simulink model "Simulink_multiterminal_HVDC_grid"  (R2016a)
settings: Solver=ode4  StartTime=0.0  StopTime=tsimul  FixedStep=1e-5  MaxStep=1e-4  RelTol=1e-5
values from neighbouring files (symbols this model uses):
  c = 0.1616*(10^-6)    (= 1.616e-07)    [Parameters_multiterminal_HVDC_grid.m]
  Cconv = 1.5*(10^-4)    (= 0.00015)    [Parameters_multiterminal_HVDC_grid.m]
  d1 = 230    [Parameters_multiterminal_HVDC_grid.m]
  d2 = 75    [Parameters_multiterminal_HVDC_grid.m]
  d3 = 217    [Parameters_multiterminal_HVDC_grid.m]
  E2ref = 640000    [Parameters_multiterminal_HVDC_grid.m]
  Kp = 0.0017    [Parameters_multiterminal_HVDC_grid.m]
  l1 = 0.2644*(10^-3)    (= 0.0002644)    [Parameters_multiterminal_HVDC_grid.m]
  l2 = 7.2865*(10^-3)    (= 0.0072865)    [Parameters_multiterminal_HVDC_grid.m]
  l3 = 3.6198*(10^-3)    (= 0.0036198)    [Parameters_multiterminal_HVDC_grid.m]
  Ll = 0.1956    [Parameters_multiterminal_HVDC_grid.m]
  Qref = 0    [Parameters_multiterminal_HVDC_grid.m]
  r1 = 0.1265    [Parameters_multiterminal_HVDC_grid.m]
  r2 = 0.1504    [Parameters_multiterminal_HVDC_grid.m]
  r3 = 0.0178    [Parameters_multiterminal_HVDC_grid.m]
  Rg = (1/g)    (= 9852216.74877)    [Parameters_multiterminal_HVDC_grid.m]
  rl = 3.072    [Parameters_multiterminal_HVDC_grid.m]
  tau = 0.001    [Parameters_multiterminal_HVDC_grid.m]
  taupll = 0.0045    [Parameters_multiterminal_HVDC_grid.m]
  Uab = 320000    [Parameters_multiterminal_HVDC_grid.m]
  Vdc = 640000    [Parameters_multiterminal_HVDC_grid.m]
undefined symbols (not defined in the file or in its folder): Kpdc
libraries: powerlib x115, simulink x4
(part 1 of 2)
settings Model: Creator=usuario  LastModifiedBy=usuario
settings DataIOCC: SaveFormat=StructureWithTime
settings DebuggingCC: AllowSymbolicDim=off
settings HardwareCC: ProdWordSize=32  ProdHWDeviceType=Specified

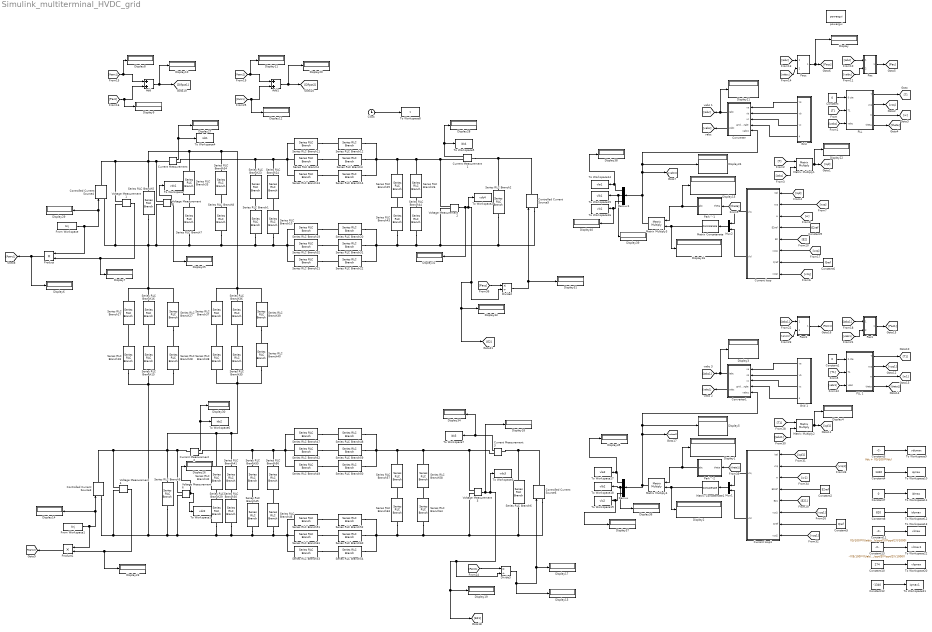
== system Simulink_multiterminal_HVDC_grid ==
  Add : Sum
  Add1 : Sum
  Clock : Clock
  Constant : Constant  Value=0
  Constant1 : Constant  Value=0
  Constant10 : Constant  Value=274
  Constant11 : Constant  Value=((5/100)*((Uab/sqrt(3))*sqrt(2))/1000)+(((Uab/sqrt(3))*sqrt(2))/1000)
  Constant12 : Constant  Value=-1340
  Constant13 : Constant  Value=-(((5/100)*((Uab/sqrt(3))*sqrt(2))/1000)+(((Uab/sqrt(3))*sqrt(2))/1000))
  Constant2 : Constant  Value=E2ref
  Constant3 : Constant  Value=Vdc + ((5/100)*Vdc)
  Constant4 : Constant  Value=1340
  Constant5 : Constant  Value=Qref
  Constant6 : Constant  Value=Qref
  Constant7 : Constant  Value=0
  Constant8 : Constant  Value=820
  Constant9 : Constant  Value=E2ref
  Controlled Current Source{3..6} (4 alike) : powerlib/Electrical Sources/Controlled Current Source  Initialize=on  Source_Type=AC  Amplitude=0  Phase=0  Frequency=0  Measurements=None
  Converter : Subsystem
  Converter1 : Subsystem
  Current Measurement{,1..3} (4 alike) : powerlib/Measurements/Current Measurement  PhasorSimulation=off  OutputType=Complex  PSBequivalent=0
  Current loop : Subsystem
  Current loop1 : Subsystem
  Demux : Demux  Outputs=3
  Demux1 : Demux  Outputs=3
  Display{,1..40} (41 alike) : Display
  Divide2 : Product  Inputs=*/
  Divide3 : Product  Inputs=*/
  From Workspace : FromWorkspace  VariableName=Iinj  SampleTime=0
  From Workspace1 : FromWorkspace  VariableName=Iinj  SampleTime=0
  "Grid " : Subsystem
  Grid 1 : Subsystem
  Matrix Concatenate : Concatenate  NumInputs=1  Mode=Multidimensional array  ConcatenateDimension=2
  Matrix Concatenate1 : Concatenate  NumInputs=1  Mode=Multidimensional array  ConcatenateDimension=2
  Matrix Multiply{1..4} (4 alike) : Product  Multiplication=Matrix(*)
  Mux1 : Mux  Inputs=2
  Mux2 : Mux  Inputs=2
  "PLL " : Subsystem
  PLL 1 : Subsystem
  Pac : Subsystem
  Pac1 : Subsystem
  Pacc : Subsystem
  Pacc1 : Subsystem
  Park^-1 : Subsystem
  Park^-2 : Subsystem
  Product : Product
  Product1 : Product
  Series RLC Branch{1,23,25,43} (4 alike) : powerlib/Elements/Series RLC Branch  LConnTagsString=__new0  RConnTagsString=__new0  BranchType=R  Resistance=(Rg/d1)*(1/2)  Inductance=1e-3  SetiL0=off  InitialCurrent=0  Capacitance=1e-6  Setx0=off  InitialVoltage=0  Measurements=None
  Series RLC Branch10 : powerlib/Elements/Series RLC Branch  LConnTagsString=__new0  RConnTagsString=__new0  BranchType=C  Resistance=0  Inductance=0  SetiL0=off  InitialCurrent=0  Capacitance=(c/2)*d1  Setx0=on  InitialVoltage=Vdc  Measurements=None
  Series RLC Branch11 : powerlib/Elements/Series RLC Branch  LConnTagsString=__new0  RConnTagsString=__new0  BranchType=R  Resistance=r1*d1  Inductance=1e-3  SetiL0=off  InitialCurrent=0  Capacitance=1e-6  Setx0=off  InitialVoltage=0  Measurements=None
  Series RLC Branch12 : powerlib/Elements/Series RLC Branch  LConnTagsString=__new0  RConnTagsString=__new0  BranchType=L  Resistance=1  Inductance=l1*d1  SetiL0=off  InitialCurrent=0  Capacitance=1e-6  Setx0=off  InitialVoltage=0  Measurements=None
  Series RLC Branch13 : powerlib/Elements/Series RLC Branch  LConnTagsString=__new0  RConnTagsString=__new0  BranchType=R  Resistance=r3*d1  Inductance=1e-3  SetiL0=off  InitialCurrent=0  Capacitance=1e-6  Setx0=off  InitialVoltage=0  Measurements=None
  Series RLC Branch14 : powerlib/Elements/Series RLC Branch  LConnTagsString=__new0  RConnTagsString=__new0  BranchType=L  Resistance=1  Inductance=l3*d1  SetiL0=off  InitialCurrent=0  Capacitance=1e-6  Setx0=off  InitialVoltage=0  Measurements=None
  Series RLC Branch15 : powerlib/Elements/Series RLC Branch  LConnTagsString=__new0  RConnTagsString=__new0  BranchType=L  Resistance=1  Inductance=l2*d2  SetiL0=off  InitialCurrent=0  Capacitance=1e-6  Setx0=off  InitialVoltage=0  Measurements=None
  Series RLC Branch16 : powerlib/Elements/Series RLC Branch  LConnTagsString=__new0  RConnTagsString=__new0  BranchType=R  Resistance=r2*d2  Inductance=1e-3  SetiL0=off  InitialCurrent=0  Capacitance=1e-6  Setx0=off  InitialVoltage=0  Measurements=None
  Series RLC Branch17 : powerlib/Elements/Series RLC Branch  LConnTagsString=__new0  RConnTagsString=__new0  BranchType=R  Resistance=r1*d2  Inductance=1e-3  SetiL0=off  InitialCurrent=0  Capacitance=1e-6  Setx0=off  InitialVoltage=0  Measurements=None
  Series RLC Branch18 : powerlib/Elements/Series RLC Branch  LConnTagsString=__new0  RConnTagsString=__new0  BranchType=L  Resistance=1  Inductance=l1*d2  SetiL0=off  InitialCurrent=0  Capacitance=1e-6  Setx0=off  InitialVoltage=0  Measurements=None
  Series RLC Branch19 : powerlib/Elements/Series RLC Branch  LConnTagsString=__new0  RConnTagsString=__new0  BranchType=R  Resistance=r1*d1  Inductance=1e-3  SetiL0=off  InitialCurrent=0  Capacitance=1e-6  Setx0=off  InitialVoltage=0  Measurements=None
  Series RLC Branch2 : powerlib/Elements/Series RLC Branch  LConnTagsString=__new0  RConnTagsString=__new0  BranchType=C  Resistance=0  Inductance=0  SetiL0=off  InitialCurrent=0  Capacitance=Cconv  Setx0=on  InitialVoltage=Vdc  Measurements=None
  Series RLC Branch20 : powerlib/Elements/Series RLC Branch  LConnTagsString=__new0  RConnTagsString=__new0  BranchType=L  Resistance=1  Inductance=l1*d1  SetiL0=off  InitialCurrent=0  Capacitance=1e-6  Setx0=off  InitialVoltage=0  Measurements=None
  Series RLC Branch21 : powerlib/Elements/Series RLC Branch  LConnTagsString=__new0  RConnTagsString=__new0  BranchType=R  Resistance=r3*d1  Inductance=1e-3  SetiL0=off  InitialCurrent=0  Capacitance=1e-6  Setx0=off  InitialVoltage=0  Measurements=None
  Series RLC Branch22 : powerlib/Elements/Series RLC Branch  LConnTagsString=__new0  RConnTagsString=__new0  BranchType=L  Resistance=1  Inductance=l3*d1  SetiL0=off  InitialCurrent=0  Capacitance=1e-6  Setx0=off  InitialVoltage=0  Measurements=None
  Series RLC Branch24 : powerlib/Elements/Series RLC Branch  LConnTagsString=__new0  RConnTagsString=__new0  BranchType=C  Resistance=0  Inductance=0  SetiL0=off  InitialCurrent=0  Capacitance=(c/2)*d1  Setx0=on  InitialVoltage=Vdc  Measurements=None
  Series RLC Branch26 : powerlib/Elements/Series RLC Branch  LConnTagsString=__new0  RConnTagsString=__new0  BranchType=C  Resistance=0  Inductance=0  SetiL0=off  InitialCurrent=0  Capacitance=(c/2)*d1  Setx0=on  InitialVoltage=Vdc  Measurements=None
  Series RLC Branch27 : powerlib/Elements/Series RLC Branch  LConnTagsString=__new0  RConnTagsString=__new0  BranchType=R  Resistance=r3*d2  Inductance=1e-3  SetiL0=off  InitialCurrent=0  Capacitance=1e-6  Setx0=off  InitialVoltage=0  Measurements=None
  Series RLC Branch28 : powerlib/Elements/Series RLC Branch  LConnTagsString=__new0  RConnTagsString=__new0  BranchType=L  Resistance=1  Inductance=l3*d2  SetiL0=off  InitialCurrent=0  Capacitance=1e-6  Setx0=off  InitialVoltage=0  Measurements=None
  Series RLC Branch29 : powerlib/Elements/Series RLC Branch  LConnTagsString=__new0  RConnTagsString=__new0  BranchType=C  Resistance=0  Inductance=0  SetiL0=off  InitialCurrent=0  Capacitance=(c/2)*d2  Setx0=on  InitialVoltage=Vdc  Measurements=None
  Series RLC Branch3 : powerlib/Elements/Series RLC Branch  LConnTagsString=__new0  RConnTagsString=__new0  BranchType=L  Resistance=1  Inductance=l2*d1  SetiL0=off  InitialCurrent=0  Capacitance=1e-6  Setx0=off  InitialVoltage=0  Measurements=None
  Series RLC Branch{7,30,33,41} (4 alike) : powerlib/Elements/Series RLC Branch  LConnTagsString=__new0  RConnTagsString=__new0  BranchType=R  Resistance=(Rg/d2)*(1/2)  Inductance=1e-3  SetiL0=off  InitialCurrent=0  Capacitance=1e-6  Setx0=off  InitialVoltage=0  Measurements=None
  Series RLC Branch31 : powerlib/Elements/Series RLC Branch  LConnTagsString=__new0  RConnTagsString=__new0  BranchType=L  Resistance=1  Inductance=l2*d1  SetiL0=off  InitialCurrent=0  Capacitance=1e-6  Setx0=off  InitialVoltage=0  Measurements=None
  Series RLC Branch32 : powerlib/Elements/Series RLC Branch  LConnTagsString=__new0  RConnTagsString=__new0  BranchType=R  Resistance=r2*d1  Inductance=1e-3  SetiL0=off  InitialCurrent=0  Capacitance=1e-6  Setx0=off  InitialVoltage=0  Measurements=None
  Series RLC Branch34 : powerlib/Elements/Series RLC Branch  LConnTagsString=__new0  RConnTagsString=__new0  BranchType=C  Resistance=0  Inductance=0  SetiL0=off  InitialCurrent=0  Capacitance=(c/2)*d2  Setx0=on  InitialVoltage=Vdc  Measurements=None
  Series RLC Branch35 : powerlib/Elements/Series RLC Branch  LConnTagsString=__new0  RConnTagsString=__new0  BranchType=L  Resistance=1  Inductance=l2*d2  SetiL0=off  InitialCurrent=0  Capacitance=1e-6  Setx0=off  InitialVoltage=0  Measurements=None
  Series RLC Branch36 : powerlib/Elements/Series RLC Branch  LConnTagsString=__new0  RConnTagsString=__new0  BranchType=R  Resistance=r2*d2  Inductance=1e-3  SetiL0=off  InitialCurrent=0  Capacitance=1e-6  Setx0=off  InitialVoltage=0  Measurements=None
  Series RLC Branch37 : powerlib/Elements/Series RLC Branch  LConnTagsString=__new0  RConnTagsString=__new0  BranchType=R  Resistance=r1*d2  Inductance=1e-3  SetiL0=off  InitialCurrent=0  Capacitance=1e-6  Setx0=off  InitialVoltage=0  Measurements=None
  Series RLC Branch38 : powerlib/Elements/Series RLC Branch  LConnTagsString=__new0  RConnTagsString=__new0  BranchType=L  Resistance=1  Inductance=l1*d2  SetiL0=off  InitialCurrent=0  Capacitance=1e-6  Setx0=off  InitialVoltage=0  Measurements=None
  Series RLC Branch39 : powerlib/Elements/Series RLC Branch  LConnTagsString=__new0  RConnTagsString=__new0  BranchType=R  Resistance=r3*d2  Inductance=1e-3  SetiL0=off  InitialCurrent=0  Capacitance=1e-6  Setx0=off  InitialVoltage=0  Measurements=None
  Series RLC Branch4 : powerlib/Elements/Series RLC Branch  LConnTagsString=__new0  RConnTagsString=__new0  BranchType=R  Resistance=r2*d1  Inductance=1e-3  SetiL0=off  InitialCurrent=0  Capacitance=1e-6  Setx0=off  InitialVoltage=0  Measurements=None
  Series RLC Branch40 : powerlib/Elements/Series RLC Branch  LConnTagsString=__new0  RConnTagsString=__new0  BranchType=L  Resistance=1  Inductance=l3*d2  SetiL0=off  InitialCurrent=0  Capacitance=1e-6  Setx0=off  InitialVoltage=0  Measurements=None
  Series RLC Branch42 : powerlib/Elements/Series RLC Branch  LConnTagsString=__new0  RConnTagsString=__new0  BranchType=C  Resistance=0  Inductance=0  SetiL0=off  InitialCurrent=0  Capacitance=(c/2)*d2  Setx0=on  InitialVoltage=Vdc  Measurements=None
  Series RLC Branch44 : powerlib/Elements/Series RLC Branch  LConnTagsString=__new0  RConnTagsString=__new0  BranchType=C  Resistance=0  Inductance=0  SetiL0=off  InitialCurrent=0  Capacitance=(c/2)*d1  Setx0=off  InitialVoltage=Vdc  Measurements=None
  Series RLC Branch{45,55,57,63} (4 alike) : powerlib/Elements/Series RLC Branch  LConnTagsString=__new0  RConnTagsString=__new0  BranchType=R  Resistance=(Rg/d3)*(1/2)  Inductance=1e-3  SetiL0=off  InitialCurrent=0  Capacitance=1e-6  Setx0=off  InitialVoltage=0  Measurements=None
  Series RLC Branch46 : powerlib/Elements/Series RLC Branch  LConnTagsString=__new0  RConnTagsString=__new0  BranchType=C  Resistance=0  Inductance=0  SetiL0=off  InitialCurrent=0  Capacitance=(c/2)*d3  Setx0=on  InitialVoltage=Vdc  Measurements=None
  Series RLC Branch47 : powerlib/Elements/Series RLC Branch  LConnTagsString=__new0  RConnTagsString=__new0  BranchType=R  Resistance=r1*d3  Inductance=1e-3  SetiL0=off  InitialCurrent=0  Capacitance=1e-6  Setx0=off  InitialVoltage=0  Measurements=None
  Series RLC Branch48 : powerlib/Elements/Series RLC Branch  LConnTagsString=__new0  RConnTagsString=__new0  BranchType=L  Resistance=1  Inductance=l1*d3  SetiL0=off  InitialCurrent=0  Capacitance=1e-6  Setx0=off  InitialVoltage=0  Measurements=None
  Series RLC Branch49 : powerlib/Elements/Series RLC Branch  LConnTagsString=__new0  RConnTagsString=__new0  BranchType=R  Resistance=r3*d3  Inductance=1e-3  SetiL0=off  InitialCurrent=0  Capacitance=1e-6  Setx0=off  InitialVoltage=0  Measurements=None
  Series RLC Branch5 : powerlib/Elements/Series RLC Branch  LConnTagsString=__new0  RConnTagsString=__new0  BranchType=C  Resistance=0  Inductance=0  SetiL0=off  InitialCurrent=0  Capacitance=Cconv  Setx0=off  InitialVoltage=Vdc  Measurements=None
  Series RLC Branch50 : powerlib/Elements/Series RLC Branch  LConnTagsString=__new0  RConnTagsString=__new0  BranchType=L  Resistance=1  Inductance=l3*d3  SetiL0=off  InitialCurrent=0  Capacitance=1e-6  Setx0=off  InitialVoltage=0  Measurements=None
  Series RLC Branch51 : powerlib/Elements/Series RLC Branch  LConnTagsString=__new0  RConnTagsString=__new0  BranchType=R  Resistance=r1*d3  Inductance=1e-3  SetiL0=off  InitialCurrent=0  Capacitance=1e-6  Setx0=off  InitialVoltage=0  Measurements=None
  Series RLC Branch52 : powerlib/Elements/Series RLC Branch  LConnTagsString=__new0  RConnTagsString=__new0  BranchType=L  Resistance=1  Inductance=l1*d3  SetiL0=off  InitialCurrent=0  Capacitance=1e-6  Setx0=off  InitialVoltage=0  Measurements=None
  Series RLC Branch53 : powerlib/Elements/Series RLC Branch  LConnTagsString=__new0  RConnTagsString=__new0  BranchType=R  Resistance=r3*d3  Inductance=1e-3  SetiL0=off  InitialCurrent=0  Capacitance=1e-6  Setx0=off  InitialVoltage=0  Measurements=None
  Series RLC Branch54 : powerlib/Elements/Series RLC Branch  LConnTagsString=__new0  RConnTagsString=__new0  BranchType=L  Resistance=1  Inductance=l3*d3  SetiL0=off  InitialCurrent=0  Capacitance=1e-6  Setx0=off  InitialVoltage=0  Measurements=None
  Series RLC Branch56 : powerlib/Elements/Series RLC Branch  LConnTagsString=__new0  RConnTagsString=__new0  BranchType=C  Resistance=0  Inductance=0  SetiL0=off  InitialCurrent=0  Capacitance=(c/2)*d3  Setx0=off  InitialVoltage=Vdc  Measurements=None
  Series RLC Branch58 : powerlib/Elements/Series RLC Branch  LConnTagsString=__new0  RConnTagsString=__new0  BranchType=C  Resistance=0  Inductance=0  SetiL0=off  InitialCurrent=0  Capacitance=(c/2)*d3  Setx0=on  InitialVoltage=Vdc  Measurements=None
  Series RLC Branch59 : powerlib/Elements/Series RLC Branch  LConnTagsString=__new0  RConnTagsString=__new0  BranchType=L  Resistance=1  Inductance=l2*d3  SetiL0=off  InitialCurrent=0  Capacitance=1e-6  Setx0=off  InitialVoltage=0  Measurements=None
  Series RLC Branch6 : powerlib/Elements/Series RLC Branch  LConnTagsString=__new0  RConnTagsString=__new0  BranchType=C  Resistance=0  Inductance=0  SetiL0=off  InitialCurrent=0  Capacitance=Cconv  Setx0=on  InitialVoltage=Vdc  Measurements=None
  Series RLC Branch60 : powerlib/Elements/Series RLC Branch  LConnTagsString=__new0  RConnTagsString=__new0  BranchType=L  Resistance=1  Inductance=l2*d3  SetiL0=off  InitialCurrent=0  Capacitance=1e-6  Setx0=off  InitialVoltage=0  Measurements=None
  Series RLC Branch61 : powerlib/Elements/Series RLC Branch  LConnTagsString=__new0  RConnTagsString=__new0  BranchType=R  Resistance=r2*d3  Inductance=1e-3  SetiL0=off  InitialCurrent=0  Capacitance=1e-6  Setx0=off  InitialVoltage=0  Measurements=None
  Series RLC Branch62 : powerlib/Elements/Series RLC Branch  LConnTagsString=__new0  RConnTagsString=__new0  BranchType=R  Resistance=r2*d3  Inductance=1e-3  SetiL0=off  InitialCurrent=0  Capacitance=1e-6  Setx0=off  InitialVoltage=0  Measurements=None
  Series RLC Branch64 : powerlib/Elements/Series RLC Branch  LConnTagsString=__new0  RConnTagsString=__new0  BranchType=C  Resistance=0  Inductance=0  SetiL0=off  InitialCurrent=0  Capacitance=(c/2)*d3  Setx0=off  InitialVoltage=Vdc  Measurements=None
  Series RLC Branch8 : powerlib/Elements/Series RLC Branch  LConnTagsString=__new0  RConnTagsString=__new0  BranchType=C  Resistance=0  Inductance=0  SetiL0=off  InitialCurrent=0  Capacitance=(c/2)*d2  Setx0=off  InitialVoltage=Vdc  Measurements=None
  Series RLC Branch9 : powerlib/Elements/Series RLC Branch  LConnTagsString=__new0  RConnTagsString=__new0  BranchType=C  Resistance=0  Inductance=0  SetiL0=off  InitialCurrent=0  Capacitance=Cconv  Setx0=off  InitialVoltage=Vdc  Measurements=None
  To Workspace : ToWorkspace  VariableName=vdc1  SampleTime=-1
  To Workspace1 : ToWorkspace  VariableName=vdc2  SampleTime=-1
  To Workspace10 : ToWorkspace  VariableName=iqmax  SampleTime=-1
  To Workspace11 : ToWorkspace  VariableName=idmax  SampleTime=-1
  To Workspace12 : ToWorkspace  VariableName=idcmax  SampleTime=-1
  To Workspace13 : ToWorkspace  VariableName=vlmax  SampleTime=-1
  To Workspace14 : ToWorkspace  VariableName=vla1  SampleTime=-1
  To Workspace15 : ToWorkspace  VariableName=vlb1  SampleTime=-1
  To Workspace16 : ToWorkspace  VariableName=vlc1  SampleTime=-1
  To Workspace17 : ToWorkspace  VariableName=vla2  SampleTime=-1
  To Workspace18 : ToWorkspace  VariableName=vlb2  SampleTime=-1
  To Workspace19 : ToWorkspace  VariableName=vlc2  SampleTime=-1
  To Workspace2 : ToWorkspace  VariableName=vdc4  SampleTime=-1
  To Workspace20 : ToWorkspace  VariableName=vlqmax  SampleTime=-1
  To Workspace21 : ToWorkspace  VariableName=iqmax1  SampleTime=-1
  To Workspace22 : ToWorkspace  VariableName=vlmax1  SampleTime=-1
  To Workspace3 : ToWorkspace  VariableName=vdc3  SampleTime=-1
  To Workspace4 : ToWorkspace  VariableName=idc1  SampleTime=-1
  To Workspace5 : ToWorkspace  VariableName=idc4  SampleTime=-1
  To Workspace6 : ToWorkspace  VariableName=idc2  SampleTime=-1
  To Workspace7 : ToWorkspace  VariableName=idc3  SampleTime=-1
  To Workspace8 : ToWorkspace  VariableName=t  SampleTime=-1
  To Workspace9 : ToWorkspace  VariableName=vdcmax  SampleTime=-1
  Voltage Measurement{1..6} (6 alike) : powerlib/Measurements/Voltage Measurement  PhasorSimulation=off  OutputType=Complex  PSBequivalent=0
  powergui : powerlib/powergui  Priority=1  SimulationMode=Continuous  SolverType=Tustin/Backward Euler (TBE)  SampleTime=50e-6  frequency=60  SPID=off  DisableSnubberDevices=off  DisableRonSwitches=off  DisableVfSwitches=off  SwTol=0  DisplayEquations=off  Interpol=off  ExternalGateDelay=off  methode=off  Ts=10  FunctionMessages=off  echomessages=off  HookPort=off  EnableUseOfTLC=off  x0status=blocks  frequencyindice=0  Pbase=100e6  ErrMax=1e-4  Iterations=50  UnitsV=kV  UnitsW=MW  buscounter=0  RestoreLinks=warning  ResistiveCurrentMeasurement=off  Frange=[0:2:500]  Ylog=off  Xlog=on  ShowGrid=off  save=off  variable=ZData  structure=0  ZoomFFT=off  StartTime=0.0  cycles=1  DisplayStyle=1  fundamental=60  FreqAxis=off  MaxFrequency=1000  frequencyindicesteady=1  RmsSteady=1  display=off
  wires:
  [T] -> Matrix Multiply1/1
  [iabc] -> Matrix Multiply1/2
  Matrix Multiply1/1 -> [iqd], Display22/1
  Park^-1/1(abc) -> Matrix Multiply3/1, Display15/1
  Matrix Multiply3/1 -> Demux1/1, Converter/5(vabcc), Display24/1, [vabcc]
  Mux2/1 -> Matrix Concatenate/1
  Matrix Concatenate/1 -> Matrix Multiply3/2, Display16/1
  [theta] -> Park^-1/1(theta)
  Constant/1 -> "PLL "/1(0 cte)
  [T] -> "PLL "/2(T1)
  [vabc] -> "PLL "/3(vabc)
  "PLL "/1(T) -> [T]
  "PLL "/2(vzq) -> [vzq]
  "PLL "/3(w) -> [w]
  "PLL "/4(theta) -> [theta]
  [iqd] -> Current loop/1(iqd)
  [vzq] -> Current loop/2(vzq)
  [w] -> Current loop/3(w)
  Constant9/1 -> Current loop/4(E2ref)
  [E2] -> Current loop/5("E2 ")
  [vzq] -> Current loop/6(vzq1)
  Constant6/1 -> Current loop/7(Qref)
  [vzq] -> Current loop/8(vzq2)
  Current loop/1(vlq) -> Mux2/1
  Current loop/2(vld) -> Mux2/2
  [iabc] -> Pacc/1(iabc)
  [vabcc] -> Pacc/2(vabcc)
  Pacc/1(Pacc) -> Display/1, [Pacc]
  [iabc] -> Pac/1(iabc)
  [vabc] -> Pac/2(vabc)
  Pac/1(Pac) -> [Pac]
  Converter/1(iabc) -> Display21/1, [iabc]
  "Grid "/1(va) -> Converter/1(va)
  "Grid "/2(vb) -> Converter/2(vb)
  "Grid "/3(vc) -> Converter/3(vc)
  "Grid "/4(grid angle) -> Converter/4(grid angle)
  Converter/2(vabc) -> [vabc]
  [T1] -> Matrix Multiply2/1
  [iabc1] -> Matrix Multiply2/2
  Matrix Multiply2/1 -> [iqd1], Display4/1
  Park^-2/1(abc) -> Matrix Multiply4/1, Display1/1
  Matrix Multiply4/1 -> Converter1/5(vabcc), Display5/1, [vabcc1], Demux/1
  Mux1/1 -> Matrix Concatenate1/1
  Matrix Concatenate1/1 -> Matrix Multiply4/2, Display2/1
  [theta1] -> Park^-2/1(theta)
  Constant1/1 -> PLL 1/1(0 cte)
  [T1] -> PLL 1/2(T1)
  [vabc1] -> PLL 1/3(vabc)
  PLL 1/1(T) -> [T1]
  PLL 1/2(vzq) -> [vzq1]
  PLL 1/3(w) -> [w1]
  PLL 1/4(theta) -> [theta1]
  [iqd1] -> Current loop1/1(iqd)
  [vzq1] -> Current loop1/2(vzq)
  [w1] -> Current loop1/3(w)
  Constant2/1 -> Current loop1/4(E2ref)
  [E21] -> Current loop1/5("E21 ")
  [vzq1] -> Current loop1/6(vzq1)
  Constant5/1 -> Current loop1/7(Qref)
  [vzq1] -> Current loop1/8(vzq2)
  Current loop1/1(vlq) -> Mux1/1
  Current loop1/2(vld) -> Mux1/2
  [iabc1] -> Pacc1/1(iabc)
  [vabcc1] -> Pacc1/2(vabcc)
  Pacc1/1(Pacc) -> [Pacc1]
  [iabc1] -> Pac1/1(iabc)
  [vabc1] -> Pac1/2(vabc)
  Pac1/1(Pac) -> [Pac1]
  Converter1/1(iabc) -> Display3/1, [iabc1]
  Grid 1/1(va) -> Converter1/1(va)
  Grid 1/2(vb) -> Converter1/2(vb)
  Grid 1/3(vc) -> Converter1/3(vc)
  Grid 1/4(grid angle) -> Converter1/4(grid angle)
  Converter1/2(vabc) -> [vabc1]
  Voltage Measurement2/1 -> Display32/1, To Workspace2/1, [E2], Display33/1, Divide2/2
  Divide2/1 -> Display31/1, Controlled Current Source5/1
  [Pacc] -> Divide2/1
  From Workspace/1 -> Product/1, Display29/1, Controlled Current Source4/1
  Voltage Measurement3/1 -> To Workspace3/1, [E21], Display19/1, Divide3/2, Display18/1
  Divide3/1 -> Display13/1, Controlled Current Source6/1, Display17/1
  [Pacc1] -> Divide3/1
  From Workspace1/1 -> Product1/1, Display14/1, Controlled Current Source3/1
  Voltage Measurement1/1 -> Display7/1, Product/2
  Product/1 -> Display6/1, [Pparc1]
  Voltage Measurement4/1 -> Display23/1, Product1/2
  Product1/1 -> [Pparc2]
  [Pparc1] -> Display8/1, Add/1
  [Pacc] -> Display9/1, Add/2
  Add/1 -> Display10/1, [Difpot1]
  [Pparc2] -> Display11/1, Add1/1
  [Pacc1] -> Display12/1, Add1/2
  Add1/1 -> Display20/1, [Difpot2]
  Voltage Measurement5/1 -> To Workspace/1, Display25/1
  Voltage Measurement6/1 -> Display26/1, To Workspace1/1
  Current Measurement/1 -> To Workspace4/1, Display27/1
  Current Measurement1/1 -> To Workspace5/1, Display28/1
  Current Measurement2/1 -> Display30/1, To Workspace6/1
  Current Measurement3/1 -> Display34/1, To Workspace7/1
  Clock/1 -> To Workspace8/1
  Constant3/1 -> To Workspace9/1
  Constant4/1 -> To Workspace10/1
  Constant7/1 -> To Workspace11/1
  Constant8/1 -> To Workspace12/1
  Demux1/1 -> Display38/1, To Workspace14/1
  Demux1/2 -> Display39/1, To Workspace15/1
  Demux1/3 -> Display40/1, To Workspace16/1
  Demux/1 -> Display35/1, To Workspace17/1
  Demux/2 -> Display36/1, To Workspace18/1
  Demux/3 -> Display37/1, To Workspace19/1
  Constant11/1 -> To Workspace13/1
  Constant10/1 -> To Workspace20/1
  Constant12/1 -> To Workspace21/1
  Constant13/1 -> To Workspace22/1
  connections:
  Series RLC Branch14/RConn1 -- Voltage Measurement2/LConn1 -- Current Measurement1/RConn1 -- Series RLC Branch26/LConn1 -- Series RLC Branch25/LConn1 -- Series RLC Branch12/RConn1 -- Series RLC Branch3/RConn1
  Series RLC Branch35/RConn1 -- Series RLC Branch36/RConn1
  Series RLC Branch39/RConn1 -- Series RLC Branch40/RConn1
  Series RLC Branch11/RConn1 -- Series RLC Branch12/LConn1
  Series RLC Branch4/RConn1 -- Series RLC Branch3/LConn1
  Series RLC Branch13/RConn1 -- Series RLC Branch14/LConn1
  Series RLC Branch38/RConn1 -- Series RLC Branch37/RConn1
  Series RLC Branch40/LConn1 -- Series RLC Branch35/LConn1 -- Series RLC Branch38/LConn1 -- Voltage Measurement6/LConn1 -- Current Measurement2/LConn1 -- Voltage Measurement4/LConn1 -- Controlled Current Source3/RConn1 -- Series RLC Branch9/LConn1 -- Series RLC Branch42/LConn1 -- Series RLC Branch41/LConn1
  Series RLC Branch13/LConn1 -- Series RLC Branch4/LConn1 -- Series RLC Branch11/LConn1 -- Series RLC Branch23/LConn1 -- Current Measurement/RConn1 -- Series RLC Branch24/LConn1
  Series RLC Branch1/LConn1 -- Series RLC Branch23/RConn1
  Series RLC Branch10/LConn1 -- Series RLC Branch24/RConn1
  Series RLC Branch31/RConn1 -- Voltage Measurement2/LConn2 -- Series RLC Branch2/RConn1 -- Controlled Current Source5/LConn1 -- Series RLC Branch44/RConn1 -- Series RLC Branch43/RConn1 -- Series RLC Branch22/RConn1 -- Series RLC Branch20/RConn1
  Series RLC Branch21/RConn1 -- Series RLC Branch22/LConn1
  Series RLC Branch32/RConn1 -- Series RLC Branch31/LConn1
  Series RLC Branch19/RConn1 -- Series RLC Branch20/LConn1
  Series RLC Branch43/LConn1 -- Series RLC Branch25/RConn1
  Series RLC Branch44/LConn1 -- Series RLC Branch26/RConn1
  Series RLC Branch59/RConn1 -- Voltage Measurement3/LConn1 -- Current Measurement3/RConn1 -- Series RLC Branch58/LConn1 -- Series RLC Branch57/LConn1 -- Series RLC Branch50/RConn1 -- Series RLC Branch48/RConn1
  Series RLC Branch60/RConn1 -- Series RLC Branch6/RConn1 -- Controlled Current Source6/LConn1 -- Voltage Measurement3/LConn2 -- Series RLC Branch64/RConn1 -- Series RLC Branch63/RConn1 -- Series RLC Branch54/RConn1 -- Series RLC Branch52/RConn1
  Series RLC Branch51/LConn1 -- Voltage Measurement6/LConn2 -- Voltage Measurement4/LConn2 -- Controlled Current Source3/LConn1 -- Series RLC Branch28/LConn1 -- Series RLC Branch18/LConn1 -- Series RLC Branch15/LConn1 -- Series RLC Branch9/RConn1 -- Series RLC Branch29/RConn1 -- Series RLC Branch30/RConn1 -- Series RLC Branch45/RConn1 -- Series RLC Branch46/RConn1 -- Series RLC Branch53/LConn1 -- Series RLC Branch61/LConn1
  Series RLC Branch63/LConn1 -- Series RLC Branch57/RConn1
  Series RLC Branch49/RConn1 -- Series RLC Branch50/LConn1
  Series RLC Branch46/LConn1 -- Series RLC Branch56/RConn1
  Series RLC Branch47/RConn1 -- Series RLC Branch48/LConn1
  Series RLC Branch64/LConn1 -- Series RLC Branch58/RConn1
  Series RLC Branch53/RConn1 -- Series RLC Branch54/LConn1
  Series RLC Branch62/RConn1 -- Series RLC Branch59/LConn1
  Series RLC Branch51/RConn1 -- Series RLC Branch52/LConn1
  Series RLC Branch45/LConn1 -- Series RLC Branch55/RConn1
  Series RLC Branch61/RConn1 -- Series RLC Branch60/LConn1
  Series RLC Branch7/LConn1 -- Series RLC Branch33/RConn1
  Series RLC Branch8/LConn1 -- Series RLC Branch34/RConn1
  Series RLC Branch1/RConn1 -- Series RLC Branch7/RConn1 -- Voltage Measurement5/LConn2 -- Series RLC Branch27/LConn1 -- Series RLC Branch17/LConn1 -- Series RLC Branch16/LConn1 -- Voltage Measurement1/LConn2 -- Controlled Current Source4/LConn1 -- Series RLC Branch5/RConn1 -- Series RLC Branch8/RConn1 -- Series RLC Branch21/LConn1 -- Series RLC Branch32/LConn1 -- Series RLC Branch19/LConn1 -- Series RLC Branch10/RConn1
  Series RLC Branch27/RConn1 -- Series RLC Branch28/RConn1
  Series RLC Branch15/RConn1 -- Series RLC Branch16/RConn1
  Series RLC Branch18/RConn1 -- Series RLC Branch17/RConn1
  Series RLC Branch29/LConn1 -- Series RLC Branch42/RConn1
  Series RLC Branch30/LConn1 -- Series RLC Branch41/RConn1
  Controlled Current Source4/RConn1 -- Voltage Measurement1/LConn1 -- Current Measurement/LConn1 -- Voltage Measurement5/LConn1 -- Series RLC Branch39/LConn1 -- Series RLC Branch37/LConn1 -- Series RLC Branch36/LConn1 -- Series RLC Branch34/LConn1 -- Series RLC Branch33/LConn1 -- Series RLC Branch5/LConn1
  Series RLC Branch2/LConn1 -- Current Measurement1/LConn1 -- Controlled Current Source5/RConn1
  Series RLC Branch49/LConn1 -- Series RLC Branch55/LConn1 -- Current Measurement2/RConn1 -- Series RLC Branch56/LConn1 -- Series RLC Branch47/LConn1 -- Series RLC Branch62/LConn1
  Controlled Current Source6/RConn1 -- Series RLC Branch6/LConn1 -- Current Measurement3/LConn1

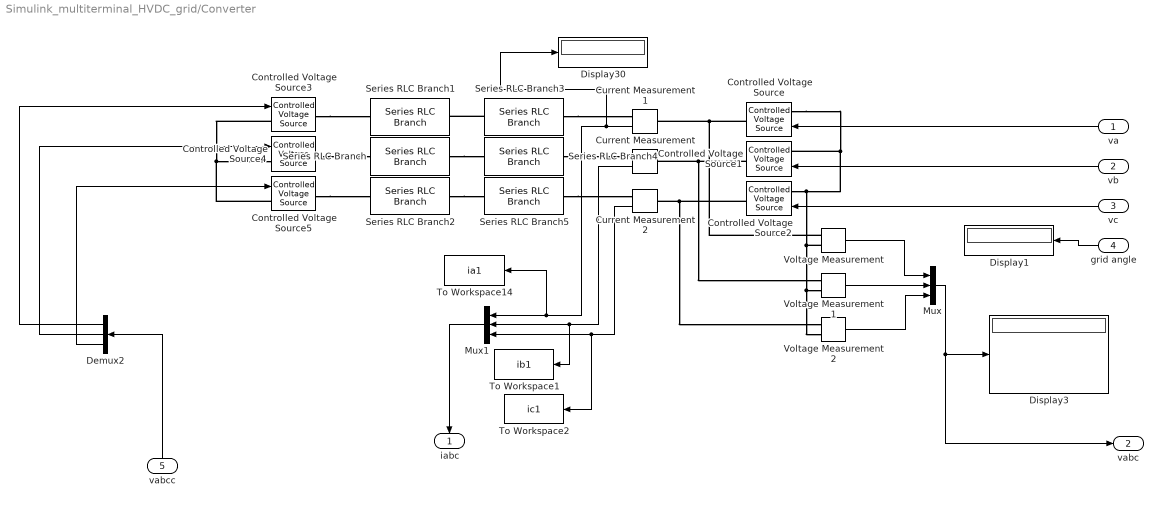
== system Simulink_multiterminal_HVDC_grid/Converter ==
  va : Inport
  vb : Inport  Port=2
  vc : Inport  Port=3
  grid angle : Inport  Port=4
  vabcc : Inport  Port=5
  Controlled Voltage Source{,1..5} (6 alike) : powerlib/Electrical Sources/Controlled Voltage Source  Initialize=on  Source_Type=AC  Amplitude=0  Phase=0  Frequency=0  Measurements=None
  Current Measurement : powerlib/Measurements/Current Measurement  PhasorSimulation=off  OutputType=Complex  PSBequivalent=0
  Current Measurement1 : powerlib/Measurements/Current Measurement  PhasorSimulation=off  OutputType=Complex  PSBequivalent=0
  Current Measurement2 : powerlib/Measurements/Current Measurement  PhasorSimulation=off  OutputType=Complex  PSBequivalent=0
  Demux2 : Demux  Outputs=3
  Display1 : Display
  Display3 : Display
  Display30 : Display
  Mux : Mux  Inputs=3
  Mux1 : Mux  Inputs=3
  Series RLC Branch : powerlib/Elements/Series RLC Branch  LConnTagsString=__new0  RConnTagsString=__new0  BranchType=R  Resistance=rl  Inductance=1e-3  SetiL0=off  InitialCurrent=0  Capacitance=1e-6  Setx0=off  InitialVoltage=0  Measurements=None
  Series RLC Branch1 : powerlib/Elements/Series RLC Branch  LConnTagsString=__new0  RConnTagsString=__new0  BranchType=R  Resistance=rl  Inductance=1e-3  SetiL0=off  InitialCurrent=0  Capacitance=1e-6  Setx0=off  InitialVoltage=0  Measurements=None
  Series RLC Branch2 : powerlib/Elements/Series RLC Branch  LConnTagsString=__new0  RConnTagsString=__new0  BranchType=R  Resistance=rl  Inductance=1e-3  SetiL0=off  InitialCurrent=0  Capacitance=1e-6  Setx0=off  InitialVoltage=0  Measurements=None
  Series RLC Branch3 : powerlib/Elements/Series RLC Branch  LConnTagsString=__new0  RConnTagsString=__new0  BranchType=L  Resistance=1  Inductance=Ll  SetiL0=off  InitialCurrent=0  Capacitance=1e-6  Setx0=off  InitialVoltage=0  Measurements=None
  Series RLC Branch4 : powerlib/Elements/Series RLC Branch  LConnTagsString=__new0  RConnTagsString=__new0  BranchType=L  Resistance=1  Inductance=Ll  SetiL0=off  InitialCurrent=0  Capacitance=1e-6  Setx0=off  InitialVoltage=0  Measurements=None
  Series RLC Branch5 : powerlib/Elements/Series RLC Branch  LConnTagsString=__new0  RConnTagsString=__new0  BranchType=L  Resistance=1  Inductance=Ll  SetiL0=off  InitialCurrent=0  Capacitance=1e-6  Setx0=off  InitialVoltage=0  Measurements=None
  To Workspace1 : ToWorkspace  VariableName=ib1  SampleTime=-1
  To Workspace14 : ToWorkspace  VariableName=ia1  SampleTime=-1
  To Workspace2 : ToWorkspace  VariableName=ic1  SampleTime=-1
  Voltage Measurement : powerlib/Measurements/Voltage Measurement  PhasorSimulation=off  OutputType=Complex  PSBequivalent=0
  Voltage Measurement1 : powerlib/Measurements/Voltage Measurement  PhasorSimulation=off  OutputType=Complex  PSBequivalent=0
  Voltage Measurement2 : powerlib/Measurements/Voltage Measurement  PhasorSimulation=off  OutputType=Complex  PSBequivalent=0
  iabc : Outport
  vabc : Outport  Port=2
  wires:
  Current Measurement1/1 -> Display30/1, To Workspace14/1, Mux1/1
  Mux1/1 -> iabc/1
  Demux2/2 -> Controlled Voltage Source4/1
  vc/1 -> Controlled Voltage Source2/1
  Demux2/3 -> Controlled Voltage Source5/1
  grid angle/1 -> Display1/1
  Voltage Measurement/1 -> Mux/1
  Demux2/1 -> Controlled Voltage Source3/1
  Mux/1 -> vabc/1, Display3/1
  Voltage Measurement2/1 -> Mux/3
  vb/1 -> Controlled Voltage Source1/1
  Current Measurement2/1 -> To Workspace2/1, Mux1/3
  va/1 -> Controlled Voltage Source/1
  Current Measurement/1 -> To Workspace1/1, Mux1/2
  Voltage Measurement1/1 -> Mux/2
  vabcc/1 -> Demux2/1
  connections:
  Series RLC Branch/RConn1 -- Series RLC Branch4/LConn1
  Controlled Voltage Source3/RConn1 -- Series RLC Branch1/LConn1
  Series RLC Branch2/RConn1 -- Series RLC Branch5/LConn1
  Controlled Voltage Source/RConn1 -- Voltage Measurement/LConn1 -- Current Measurement1/LConn1
  Series RLC Branch3/LConn1 -- Series RLC Branch1/RConn1
  Series RLC Branch3/RConn1 -- Current Measurement1/RConn1
  Controlled Voltage Source1/RConn1 -- Current Measurement/LConn1 -- Voltage Measurement1/LConn1
  Controlled Voltage Source5/RConn1 -- Series RLC Branch2/LConn1
  Series RLC Branch4/RConn1 -- Current Measurement/RConn1
  Controlled Voltage Source/LConn1 -- Controlled Voltage Source2/LConn1 -- Voltage Measurement/LConn2 -- Voltage Measurement1/LConn2 -- Voltage Measurement2/LConn2 -- Controlled Voltage Source1/LConn1
  Series RLC Branch5/RConn1 -- Current Measurement2/RConn1
  Controlled Voltage Source3/LConn1 -- Controlled Voltage Source5/LConn1 -- Controlled Voltage Source4/LConn1
  Controlled Voltage Source2/RConn1 -- Current Measurement2/LConn1 -- Voltage Measurement2/LConn1
  Controlled Voltage Source4/RConn1 -- Series RLC Branch/LConn1

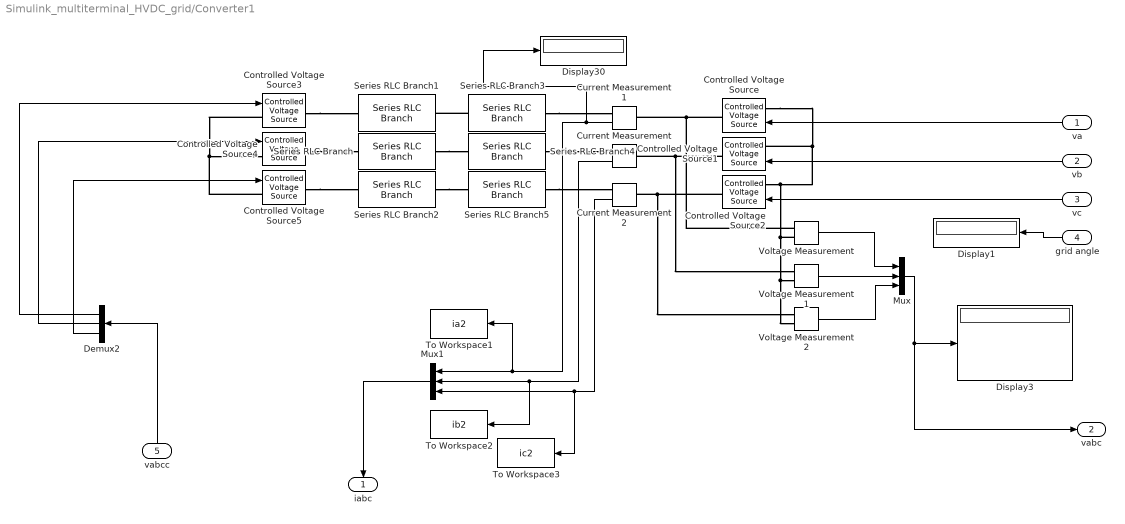
== system Simulink_multiterminal_HVDC_grid/Converter1 ==
  va : Inport
  vb : Inport  Port=2
  vc : Inport  Port=3
  grid angle : Inport  Port=4
  vabcc : Inport  Port=5
  Controlled Voltage Source{,1..5} (6 alike) : powerlib/Electrical Sources/Controlled Voltage Source  Initialize=on  Source_Type=AC  Amplitude=0  Phase=0  Frequency=0  Measurements=None
  Current Measurement : powerlib/Measurements/Current Measurement  PhasorSimulation=off  OutputType=Complex  PSBequivalent=0
  Current Measurement1 : powerlib/Measurements/Current Measurement  PhasorSimulation=off  OutputType=Complex  PSBequivalent=0
  Current Measurement2 : powerlib/Measurements/Current Measurement  PhasorSimulation=off  OutputType=Complex  PSBequivalent=0
  Demux2 : Demux  Outputs=3
  Display1 : Display
  Display3 : Display
  Display30 : Display
  Mux : Mux  Inputs=3
  Mux1 : Mux  Inputs=3
  Series RLC Branch : powerlib/Elements/Series RLC Branch  LConnTagsString=__new0  RConnTagsString=__new0  BranchType=R  Resistance=rl  Inductance=1e-3  SetiL0=off  InitialCurrent=0  Capacitance=1e-6  Setx0=off  InitialVoltage=0  Measurements=None
  Series RLC Branch1 : powerlib/Elements/Series RLC Branch  LConnTagsString=__new0  RConnTagsString=__new0  BranchType=R  Resistance=rl  Inductance=1e-3  SetiL0=off  InitialCurrent=0  Capacitance=1e-6  Setx0=off  InitialVoltage=0  Measurements=None
  Series RLC Branch2 : powerlib/Elements/Series RLC Branch  LConnTagsString=__new0  RConnTagsString=__new0  BranchType=R  Resistance=rl  Inductance=1e-3  SetiL0=off  InitialCurrent=0  Capacitance=1e-6  Setx0=off  InitialVoltage=0  Measurements=None
  Series RLC Branch3 : powerlib/Elements/Series RLC Branch  LConnTagsString=__new0  RConnTagsString=__new0  BranchType=L  Resistance=1  Inductance=Ll  SetiL0=off  InitialCurrent=0  Capacitance=1e-6  Setx0=off  InitialVoltage=0  Measurements=None
  Series RLC Branch4 : powerlib/Elements/Series RLC Branch  LConnTagsString=__new0  RConnTagsString=__new0  BranchType=L  Resistance=1  Inductance=Ll  SetiL0=off  InitialCurrent=0  Capacitance=1e-6  Setx0=off  InitialVoltage=0  Measurements=None
  Series RLC Branch5 : powerlib/Elements/Series RLC Branch  LConnTagsString=__new0  RConnTagsString=__new0  BranchType=L  Resistance=1  Inductance=Ll  SetiL0=off  InitialCurrent=0  Capacitance=1e-6  Setx0=off  InitialVoltage=0  Measurements=None
  To Workspace1 : ToWorkspace  VariableName=ia2  SampleTime=-1
  To Workspace2 : ToWorkspace  VariableName=ib2  SampleTime=-1
  To Workspace3 : ToWorkspace  VariableName=ic2  SampleTime=-1
  Voltage Measurement : powerlib/Measurements/Voltage Measurement  PhasorSimulation=off  OutputType=Complex  PSBequivalent=0
  Voltage Measurement1 : powerlib/Measurements/Voltage Measurement  PhasorSimulation=off  OutputType=Complex  PSBequivalent=0
  Voltage Measurement2 : powerlib/Measurements/Voltage Measurement  PhasorSimulation=off  OutputType=Complex  PSBequivalent=0
  iabc : Outport
  vabc : Outport  Port=2
  wires:
  Current Measurement1/1 -> Display30/1, To Workspace1/1, Mux1/1
  Mux1/1 -> iabc/1
  Demux2/2 -> Controlled Voltage Source4/1
  vc/1 -> Controlled Voltage Source2/1
  Demux2/3 -> Controlled Voltage Source5/1
  grid angle/1 -> Display1/1
  Voltage Measurement/1 -> Mux/1
  Demux2/1 -> Controlled Voltage Source3/1
  Mux/1 -> vabc/1, Display3/1
  Voltage Measurement2/1 -> Mux/3
  vb/1 -> Controlled Voltage Source1/1
  Current Measurement2/1 -> To Workspace3/1, Mux1/3
  va/1 -> Controlled Voltage Source/1
  Current Measurement/1 -> To Workspace2/1, Mux1/2
  Voltage Measurement1/1 -> Mux/2
  vabcc/1 -> Demux2/1
  connections:
  Series RLC Branch/RConn1 -- Series RLC Branch4/LConn1
  Controlled Voltage Source3/RConn1 -- Series RLC Branch1/LConn1
  Series RLC Branch2/RConn1 -- Series RLC Branch5/LConn1
  Controlled Voltage Source/RConn1 -- Voltage Measurement/LConn1 -- Current Measurement1/LConn1
  Series RLC Branch3/LConn1 -- Series RLC Branch1/RConn1
  Series RLC Branch3/RConn1 -- Current Measurement1/RConn1
  Controlled Voltage Source1/RConn1 -- Current Measurement/LConn1 -- Voltage Measurement1/LConn1
  Controlled Voltage Source5/RConn1 -- Series RLC Branch2/LConn1
  Series RLC Branch4/RConn1 -- Current Measurement/RConn1
  Controlled Voltage Source/LConn1 -- Controlled Voltage Source2/LConn1 -- Voltage Measurement/LConn2 -- Voltage Measurement1/LConn2 -- Voltage Measurement2/LConn2 -- Controlled Voltage Source1/LConn1
  Series RLC Branch5/RConn1 -- Current Measurement2/RConn1
  Controlled Voltage Source3/LConn1 -- Controlled Voltage Source5/LConn1 -- Controlled Voltage Source4/LConn1
  Controlled Voltage Source2/RConn1 -- Current Measurement2/LConn1 -- Voltage Measurement2/LConn1
  Controlled Voltage Source4/RConn1 -- Series RLC Branch/LConn1

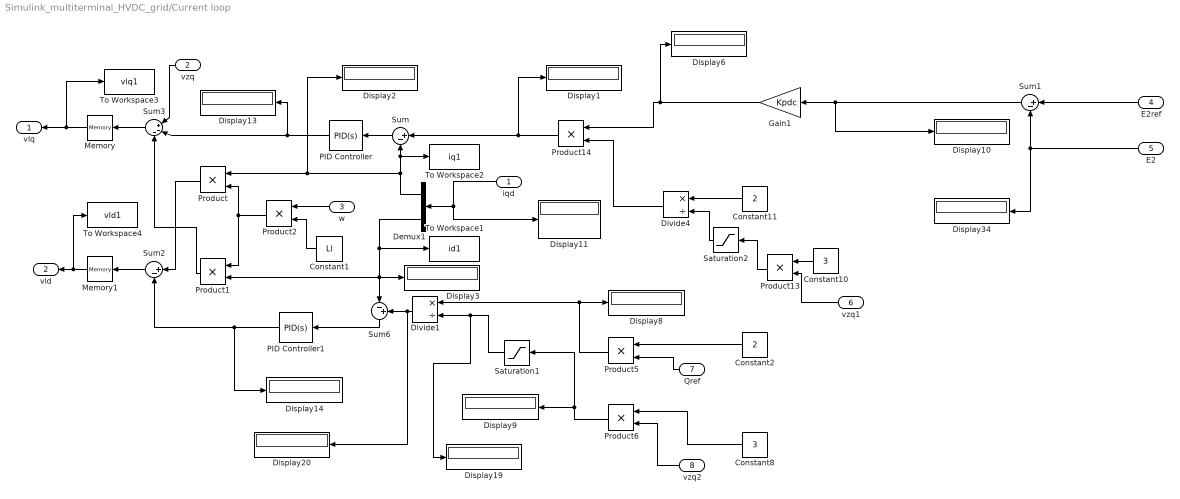
== system Simulink_multiterminal_HVDC_grid/Current loop ==
  iqd : Inport
  vzq : Inport  Port=2
  w : Inport  Port=3
  E2ref : Inport  Port=4
  "E2 " : Inport  Port=5
  vzq1 : Inport  Port=6
  Qref : Inport  Port=7
  vzq2 : Inport  Port=8
  Constant1 : Constant  Value=Ll
  Constant10 : Constant  Value=3
  Constant11 : Constant  Value=2
  Constant2 : Constant  Value=2
  Constant8 : Constant  Value=3
  Demux1 : Demux  Outputs=2
  Display{1..3,6,8..11,13..14,19..20,34} (13 alike) : Display
  Divide1 : Product  Inputs=*/
  Divide4 : Product  Inputs=*/
  Gain1 : Gain  Gain=Kpdc
  Memory : Memory
  Memory1 : Memory
  PID Controller : simulink/Continuous/PID Controller  Controller=PID  TimeDomain=Continuous-time  SampleTime=-1  IntegratorMethod=Forward Euler  FilterMethod=Forward Euler  Form=Parallel  UseFilter=on  ControllerParametersSource=internal  P=Ll/tau  I=rl/tau  D=0  N=100  InitialConditionSource=internal  InitialConditionForIntegrator=0  InitialConditionForFilter=0  ExternalReset=none  LimitOutput=off  UpperSaturationLimit=inf  LowerSaturationLimit=-inf  LinearizeAsGain=on  AntiWindupMode=none  Kb=1  TrackingMode=off  Kt=1  PParamMin=[]  PParamMax=[]  IParamMin=[]  IParamMax=[]  DParamMin=[]  DParamMax=[]  NParamMin=[]  NParamMax=[]  KbParamMin=[]  KbParamMax=[]  KtParamMin=[]  KtParamMax=[]  POutMin=[]  POutMax=[]  IOutMin=[]  IOutMax=[]  DOutMin=[]  DOutMax=[]  NOutMin=[]  NOutMax=[]  KbOutMin=[]  KbOutMax=[]  KtOutMin=[]  KtOutMax=[]  IntegratorOutMin=[]  IntegratorOutMax=[]  FilterOutMin=[]  FilterOutMax=[]  SumOutMin=[]  SumOutMax=[]  SumI1OutMin=[]  SumI1OutMax=[]  SumI2OutMin=[]  SumI2OutMax=[]  SumI3OutMin=[]  SumI3OutMax=[]  SumDOutMin=[]  SumDOutMax=[]  SaturationOutMin=[]  SaturationOutMax=[]  IntegratorContinuousStateAttributes=''  IntegratorStateMustResolveToSignalObject=off  IntegratorRTWStateStorageClass=Auto  FilterContinuousStateAttributes=''  FilterStateMustResolveToSignalObject=off  FilterRTWStateStorageClass=Auto  DifferentiatorICPrevScaledInput=0  DifferentiatorOutMin=[]  DifferentiatorOutMax=[]
  PID Controller1 : simulink/Continuous/PID Controller  Controller=PID  TimeDomain=Continuous-time  SampleTime=-1  IntegratorMethod=Forward Euler  FilterMethod=Forward Euler  Form=Parallel  UseFilter=on  ControllerParametersSource=internal  P=Ll/tau  I=rl/tau  D=0  N=100  InitialConditionSource=internal  InitialConditionForIntegrator=0  InitialConditionForFilter=0  ExternalReset=none  LimitOutput=off  UpperSaturationLimit=inf  LowerSaturationLimit=-inf  LinearizeAsGain=on  AntiWindupMode=none  Kb=1  TrackingMode=off  Kt=1  PParamMin=[]  PParamMax=[]  IParamMin=[]  IParamMax=[]  DParamMin=[]  DParamMax=[]  NParamMin=[]  NParamMax=[]  KbParamMin=[]  KbParamMax=[]  KtParamMin=[]  KtParamMax=[]  POutMin=[]  POutMax=[]  IOutMin=[]  IOutMax=[]  DOutMin=[]  DOutMax=[]  NOutMin=[]  NOutMax=[]  KbOutMin=[]  KbOutMax=[]  KtOutMin=[]  KtOutMax=[]  IntegratorOutMin=[]  IntegratorOutMax=[]  FilterOutMin=[]  FilterOutMax=[]  SumOutMin=[]  SumOutMax=[]  SumI1OutMin=[]  SumI1OutMax=[]  SumI2OutMin=[]  SumI2OutMax=[]  SumI3OutMin=[]  SumI3OutMax=[]  SumDOutMin=[]  SumDOutMax=[]  SaturationOutMin=[]  SaturationOutMax=[]  IntegratorContinuousStateAttributes=''  IntegratorStateMustResolveToSignalObject=off  IntegratorRTWStateStorageClass=Auto  FilterContinuousStateAttributes=''  FilterStateMustResolveToSignalObject=off  FilterRTWStateStorageClass=Auto  DifferentiatorICPrevScaledInput=0  DifferentiatorOutMin=[]  DifferentiatorOutMax=[]
  Product{,1..2,5..6,13..14} (7 alike) : Product
  Saturation1 : Saturate  UpperLimit=100000000000  LowerLimit=200
  Saturation2 : Saturate  UpperLimit=1000000000  LowerLimit=200
  Sum : Sum  Inputs=|+-
  Sum1 : Sum  Inputs=|+-
  Sum2 : Sum  Inputs=|+-
  Sum3 : Sum  Inputs=|+--
  Sum6 : Sum  Inputs=|-+
  To Workspace1 : ToWorkspace  VariableName=id1  SampleTime=-1
  To Workspace2 : ToWorkspace  VariableName=iq1  SampleTime=-1
  To Workspace3 : ToWorkspace  VariableName=vlq1  SampleTime=-1
  To Workspace4 : ToWorkspace  VariableName=vld1  SampleTime=-1
  vlq : Outport
  vld : Outport  Port=2
  wires:
  Constant1/1 -> Product2/2
  Qref/1 -> Product5/2
  Saturation1/1 -> Display19/1, Divide1/2
  w/1 -> Product2/1
  Product1/1 -> Sum3/3
  Demux1/2 -> To Workspace1/1, Display3/1, Sum6/1, Product1/2
  Demux1/1 -> To Workspace2/1, Sum/2, Display2/1, Product/1
  Product6/1 -> Saturation1/1, Display9/1
  PID Controller/1 -> Sum3/2, Display13/1
  PID Controller1/1 -> Sum2/2, Display14/1
  iqd/1 -> Demux1/1, Display11/1
  Sum3/1 -> Memory/1
  Product5/1 -> Divide1/1, Display8/1
  Sum2/1 -> Memory1/1
  vzq2/1 -> Product6/2
  Sum/1 -> PID Controller/1
  vzq/1 -> Sum3/1
  Product2/1 -> Product1/1, Product/2
  Divide1/1 -> Sum6/2, Display20/1
  Sum6/1 -> PID Controller1/1
  Constant8/1 -> Product6/1
  Constant2/1 -> Product5/1
  Product/1 -> Sum2/1
  Constant11/1 -> Divide4/1
  Divide4/1 -> Product14/2
  Gain1/1 -> Display6/1, Product14/1
  Sum1/1 -> Display10/1, Gain1/1
  Constant10/1 -> Product13/1
  Product13/1 -> Saturation2/1
  E2ref/1 -> Sum1/1
  "E2 "/1 -> Display34/1, Sum1/2
  Product14/1 -> Display1/1, Sum/1
  Saturation2/1 -> Divide4/2
  vzq1/1 -> Product13/2
  Memory/1 -> To Workspace3/1, vlq/1
  Memory1/1 -> To Workspace4/1, vld/1

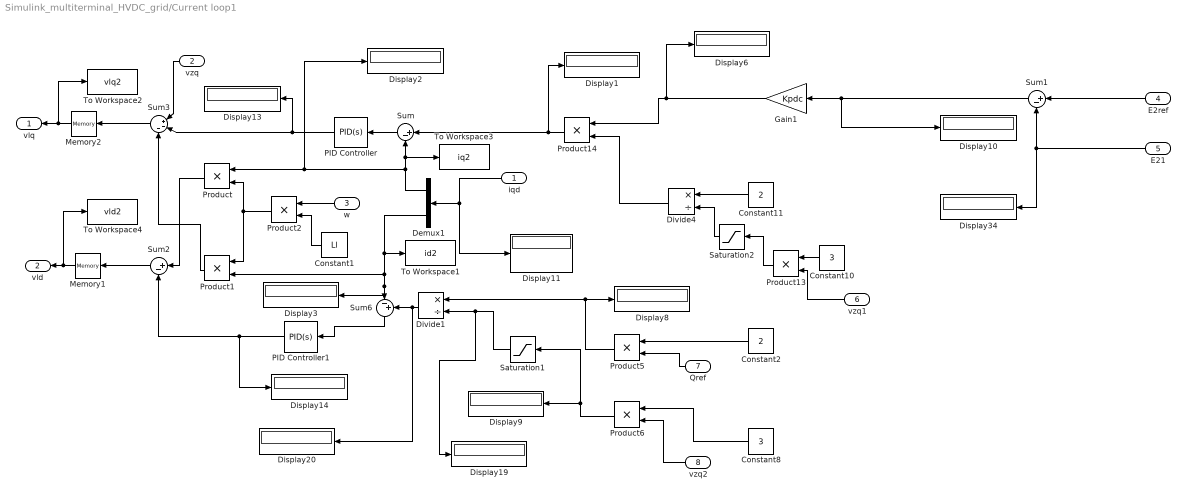
== system Simulink_multiterminal_HVDC_grid/Current loop1 ==
  iqd : Inport
  vzq : Inport  Port=2
  w : Inport  Port=3
  E2ref : Inport  Port=4
  "E21 " : Inport  Port=5
  vzq1 : Inport  Port=6
  Qref : Inport  Port=7
  vzq2 : Inport  Port=8
  Constant1 : Constant  Value=Ll
  Constant10 : Constant  Value=3
  Constant11 : Constant  Value=2
  Constant2 : Constant  Value=2
  Constant8 : Constant  Value=3
  Demux1 : Demux  Outputs=2
  Display{1..3,6,8..11,13..14,19..20,34} (13 alike) : Display
  Divide1 : Product  Inputs=*/
  Divide4 : Product  Inputs=*/
  Gain1 : Gain  Gain=Kpdc
  Memory1 : Memory
  Memory2 : Memory
  PID Controller : simulink/Continuous/PID Controller  Controller=PID  TimeDomain=Continuous-time  SampleTime=-1  IntegratorMethod=Forward Euler  FilterMethod=Forward Euler  Form=Parallel  UseFilter=on  ControllerParametersSource=internal  P=Ll/tau  I=rl/tau  D=0  N=100  InitialConditionSource=internal  InitialConditionForIntegrator=0  InitialConditionForFilter=0  ExternalReset=none  LimitOutput=off  UpperSaturationLimit=inf  LowerSaturationLimit=-inf  LinearizeAsGain=on  AntiWindupMode=none  Kb=1  TrackingMode=off  Kt=1  PParamMin=[]  PParamMax=[]  IParamMin=[]  IParamMax=[]  DParamMin=[]  DParamMax=[]  NParamMin=[]  NParamMax=[]  KbParamMin=[]  KbParamMax=[]  KtParamMin=[]  KtParamMax=[]  POutMin=[]  POutMax=[]  IOutMin=[]  IOutMax=[]  DOutMin=[]  DOutMax=[]  NOutMin=[]  NOutMax=[]  KbOutMin=[]  KbOutMax=[]  KtOutMin=[]  KtOutMax=[]  IntegratorOutMin=[]  IntegratorOutMax=[]  FilterOutMin=[]  FilterOutMax=[]  SumOutMin=[]  SumOutMax=[]  SumI1OutMin=[]  SumI1OutMax=[]  SumI2OutMin=[]  SumI2OutMax=[]  SumI3OutMin=[]  SumI3OutMax=[]  SumDOutMin=[]  SumDOutMax=[]  SaturationOutMin=[]  SaturationOutMax=[]  IntegratorContinuousStateAttributes=''  IntegratorStateMustResolveToSignalObject=off  IntegratorRTWStateStorageClass=Auto  FilterContinuousStateAttributes=''  FilterStateMustResolveToSignalObject=off  FilterRTWStateStorageClass=Auto  DifferentiatorICPrevScaledInput=0  DifferentiatorOutMin=[]  DifferentiatorOutMax=[]
  PID Controller1 : simulink/Continuous/PID Controller  Controller=PID  TimeDomain=Continuous-time  SampleTime=-1  IntegratorMethod=Forward Euler  FilterMethod=Forward Euler  Form=Parallel  UseFilter=on  ControllerParametersSource=internal  P=Ll/tau  I=rl/tau  D=0  N=100  InitialConditionSource=internal  InitialConditionForIntegrator=0  InitialConditionForFilter=0  ExternalReset=none  LimitOutput=off  UpperSaturationLimit=inf  LowerSaturationLimit=-inf  LinearizeAsGain=on  AntiWindupMode=none  Kb=1  TrackingMode=off  Kt=1  PParamMin=[]  PParamMax=[]  IParamMin=[]  IParamMax=[]  DParamMin=[]  DParamMax=[]  NParamMin=[]  NParamMax=[]  KbParamMin=[]  KbParamMax=[]  KtParamMin=[]  KtParamMax=[]  POutMin=[]  POutMax=[]  IOutMin=[]  IOutMax=[]  DOutMin=[]  DOutMax=[]  NOutMin=[]  NOutMax=[]  KbOutMin=[]  KbOutMax=[]  KtOutMin=[]  KtOutMax=[]  IntegratorOutMin=[]  IntegratorOutMax=[]  FilterOutMin=[]  FilterOutMax=[]  SumOutMin=[]  SumOutMax=[]  SumI1OutMin=[]  SumI1OutMax=[]  SumI2OutMin=[]  SumI2OutMax=[]  SumI3OutMin=[]  SumI3OutMax=[]  SumDOutMin=[]  SumDOutMax=[]  SaturationOutMin=[]  SaturationOutMax=[]  IntegratorContinuousStateAttributes=''  IntegratorStateMustResolveToSignalObject=off  IntegratorRTWStateStorageClass=Auto  FilterContinuousStateAttributes=''  FilterStateMustResolveToSignalObject=off  FilterRTWStateStorageClass=Auto  DifferentiatorICPrevScaledInput=0  DifferentiatorOutMin=[]  DifferentiatorOutMax=[]
  Product{,1..2,5..6,13..14} (7 alike) : Product
  Saturation1 : Saturate  UpperLimit=10000000000000  LowerLimit=200
  Saturation2 : Saturate  UpperLimit=1000000000000  LowerLimit=200
  Sum : Sum  Inputs=|+-
  Sum1 : Sum  Inputs=|+-
  Sum2 : Sum  Inputs=|+-
  Sum3 : Sum  Inputs=|+--
  Sum6 : Sum  Inputs=|-+
  To Workspace1 : ToWorkspace  VariableName=id2  SampleTime=-1
  To Workspace2 : ToWorkspace  VariableName=vlq2  SampleTime=-1
  To Workspace3 : ToWorkspace  VariableName=iq2  SampleTime=-1
  To Workspace4 : ToWorkspace  VariableName=vld2  SampleTime=-1
  vlq : Outport
  vld : Outport  Port=2
  wires:
  Constant1/1 -> Product2/2
  Qref/1 -> Product5/2
  Saturation1/1 -> Display19/1, Divide1/2
  w/1 -> Product2/1
  Product1/1 -> Sum3/3
  Demux1/2 -> Display3/1, Sum6/1, Product1/2, To Workspace1/1
  Demux1/1 -> Display2/1, Product/1, To Workspace3/1, Sum/2
  Product6/1 -> Saturation1/1, Display9/1
  PID Controller/1 -> Sum3/2, Display13/1
  PID Controller1/1 -> Sum2/2, Display14/1
  iqd/1 -> Demux1/1, Display11/1
  Sum3/1 -> Memory2/1
  Product5/1 -> Divide1/1, Display8/1
  Sum2/1 -> Memory1/1
  vzq2/1 -> Product6/2
  Sum/1 -> PID Controller/1
  vzq/1 -> Sum3/1
  Product2/1 -> Product1/1, Product/2
  Divide1/1 -> Sum6/2, Display20/1
  Sum6/1 -> PID Controller1/1
  Constant8/1 -> Product6/1
  Constant2/1 -> Product5/1
  Product/1 -> Sum2/1
  Constant11/1 -> Divide4/1
  Divide4/1 -> Product14/2
  Gain1/1 -> Display6/1, Product14/1
  Sum1/1 -> Display10/1, Gain1/1
  Constant10/1 -> Product13/1
  Product13/1 -> Saturation2/1
  E2ref/1 -> Sum1/1
  "E21 "/1 -> Display34/1, Sum1/2
  Product14/1 -> Display1/1, Sum/1
  Saturation2/1 -> Divide4/2
  vzq1/1 -> Product13/2
  Memory1/1 -> To Workspace4/1, vld/1
  Memory2/1 -> To Workspace2/1, vlq/1
